simulink model "e"  (R2018b)
settings: Solver=FixedStepAuto  StartTime=0.0  StopTime=10.68  FixedStep=0.01  RelTol=1e-3
settings Model: Creator=yizha  LastModifiedBy=yizha

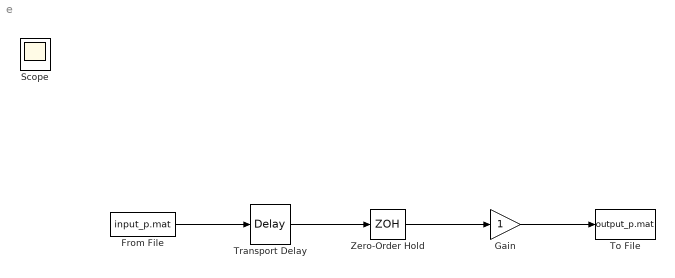
== system e ==
  From File : FromFile  FileName=input_p.mat  SampleTime=0
  Gain : Gain
  To File : ToFile  Filename=output_p.mat
  Transport Delay : TransportDelay  DelayTime=0.1
  Zero-Order Hold : ZeroOrderHold  SampleTime=0.1
  Scope : Scope
  wires:
  Gain/1 -> To File/1
  From File/1 -> Transport Delay/1
  Zero-Order Hold/1 -> Gain/1
  Transport Delay/1 -> Zero-Order Hold/1
